simulink model "my_model"  (R2025b)
settings: Solver=FixedStepAuto  StartTime=0.0  StopTime=10.0  RelTol=1e-3
model workspace (MAT data in the model file):
  net = dlnetwork
  net.any.Version = 6
  net.any.LayerGraph = nnet.cnn.LayerGraph
  net.any.LayerGraph.any.Version = 1
  net.any.LayerGraph.any.Layers(1) = nnet.cnn.layer.FeatureInputLayer
  net.any.LayerGraph.any.Layers(1).any.Version = 2
  net.any.LayerGraph.any.Layers(1).any.Name = 'input_2'
  net.any.LayerGraph.any.Layers(1).any.InputSize = 5
  net.any.LayerGraph.any.Layers(1).any.Normalization = []
  net.any.LayerGraph.any.Layers(1).any.NormalizationDimension = 'auto'
  net.any.LayerGraph.any.Layers(1).any.SplitComplexInputs = 0
  net.any.LayerGraph.any.Layers(2) = nnet.cnn.layer.FullyConnectedLayer
  net.any.LayerGraph.any.Layers(2).any.Version = 3
  net.any.LayerGraph.any.Layers(2).any.Name = 'fc_'
  net.any.LayerGraph.any.Layers(2).any.InputSize = []
  net.any.LayerGraph.any.Layers(2).any.OutputSize = 128
  net.any.LayerGraph.any.Layers(2).any.Weights.Version = 2
  net.any.LayerGraph.any.Layers(2).any.Weights.Value = [0.145622700453 0.191488698125 1.34471386946e-25 0.192500352859 7.4865119314e-32 -1.01806771917e-35 0.0375644490123 0.00493536377326 0.148149654269 0.159106627107 3.70517046692e-39 0.172035083175 ... (640 elements, 128x5)]
  net.any.LayerGraph.any.Layers(2).any.Weights.LearnRateFactor = 1
  net.any.LayerGraph.any.Layers(2).any.Weights.L2Factor = 1
  net.any.LayerGraph.any.Layers(2).any.Weights.Initializer.Version = 1
  net.any.LayerGraph.any.Layers(2).any.Weights.Initializer.Class = 'nnet.internal.cnn.layer.learnable.initializer.Glorot'
  net.any.LayerGraph.any.Layers(2).any.Weights.Initializer.ConstructorArguments = {2, 1}
  net.any.LayerGraph.any.Layers(2).any.Bias.Version = 2
  net.any.LayerGraph.any.Layers(2).any.Bias.Value = [0.0191323123872 0.0192945022136 -0.0195418279618 0.0191192030907 -7.60889611815e-15 -9.2298071408e-09 0.223294004798 -0.0135857854038 -0.0391458682716 -0.0272029154003 -0.0109884552658 -0.0147490501404 ... (128 elements, 128x1)]
  net.any.LayerGraph.any.Layers(2).any.Bias.LearnRateFactor = 1
  net.any.LayerGraph.any.Layers(2).any.Bias.L2Factor = 0
  net.any.LayerGraph.any.Layers(2).any.Bias.Initializer.Version = 1
  net.any.LayerGraph.any.Layers(2).any.Bias.Initializer.Class = 'nnet.internal.cnn.layer.learnable.initializer.Zeros'
  net.any.LayerGraph.any.Layers(2).any.Bias.Initializer.ConstructorArguments = []
  net.any.LayerGraph.any.Layers(3) = nnet.cnn.layer.ReLULayer
  net.any.LayerGraph.any.Layers(3).any.Version = 1
  net.any.LayerGraph.any.Layers(3).any.Name = 're_lu_1'
  net.any.LayerGraph.any.Layers(4) = nnet.cnn.layer.FullyConnectedLayer
  net.any.LayerGraph.any.Layers(4).any.Version = 3
  net.any.LayerGraph.any.Layers(4).any.Name = 'fc_1_'
  net.any.LayerGraph.any.Layers(4).any.InputSize = []
  net.any.LayerGraph.any.Layers(4).any.OutputSize = 1
  net.any.LayerGraph.any.Layers(4).any.Weights.Version = 2
  net.any.LayerGraph.any.Layers(4).any.Weights.Value = [0.0540892928839 0.0813860446215 3.33540966394e-25 0.0615750215948 -1.09811353254e-30 -1.90163106556e-31 0.321531116962 -0.0607957392931 -0.1230366081 -0.0873386785388 4.04759007811e-38 -0.0916871502995 ... (128 elements, 1x128)]
  net.any.LayerGraph.any.Layers(4).any.Weights.LearnRateFactor = 1
  net.any.LayerGraph.any.Layers(4).any.Weights.L2Factor = 1
  net.any.LayerGraph.any.Layers(4).any.Weights.Initializer.Version = 1
  net.any.LayerGraph.any.Layers(4).any.Weights.Initializer.Class = 'nnet.internal.cnn.layer.learnable.initializer.Glorot'
  net.any.LayerGraph.any.Layers(4).any.Weights.Initializer.ConstructorArguments = {2, 1}
  net.any.LayerGraph.any.Layers(4).any.Bias.Version = 2
  net.any.LayerGraph.any.Layers(4).any.Bias.Value = 0.0196929574013
  net.any.LayerGraph.any.Layers(4).any.Bias.LearnRateFactor = 1
  net.any.LayerGraph.any.Layers(4).any.Bias.L2Factor = 0
  net.any.LayerGraph.any.Layers(4).any.Bias.Initializer.Version = 1
  net.any.LayerGraph.any.Layers(4).any.Bias.Initializer.Class = 'nnet.internal.cnn.layer.learnable.initializer.Zeros'
  net.any.LayerGraph.any.Layers(4).any.Bias.Initializer.ConstructorArguments = []
  net.any.LayerGraph.any.Connections = table
  net.any.LayerGraph.any.Connections.data = {{'input_2'; 'fc_'; 're_lu_1'}, {'fc_'; 're_lu_1'; 'fc_1_'}}
  net.any.LayerGraph.any.Connections.ndims = 2
  net.any.LayerGraph.any.Connections.nrows = 3
  net.any.LayerGraph.any.Connections.nvars = 2
  net.any.LayerGraph.any.Connections.varnames = {'Source', 'Destination'}
  net.any.LayerGraph.any.Connections.props.CustomProps = struct()
  net.any.LayerGraph.any.Connections.props.VariableCustomProps = struct()
  net.any.LayerGraph.any.Connections.props.versionSavedFrom = 5
  net.any.LayerGraph.any.Connections.props.minCompatibleVersion = 1
  net.any.LayerGraph.any.Connections.props.incompatibilityMsg = ''
  net.any.LayerGraph.any.Connections.props.VersionSavedFrom = 5
  net.any.LayerGraph.any.Connections.props.useVariableNamesOriginal = 0
  net.any.LayerGraph.any.Connections.props.useVariableNames2048 = 0
  net.any.LayerGraph.any.Connections.props.useDimensionNamesOriginal = 0
  net.any.LayerGraph.any.Connections.props.useDimensionNames2048 = 0
  net.any.LayerGraph.any.Connections.props.Description = ''
  net.any.LayerGraph.any.Connections.props.VariableNamesOriginal = {}
  net.any.LayerGraph.any.Connections.props.VariableNames2048 = {}
  net.any.LayerGraph.any.Connections.props.DimensionNames = {'Row', 'Variables'}
  net.any.LayerGraph.any.Connections.props.DimensionNamesOriginal = {}
  net.any.LayerGraph.any.Connections.props.DimensionNames2048 = {}
  net.any.LayerGraph.any.Connections.props.UserData = []
  net.any.LayerGraph.any.Connections.props.VariableDescriptions = {}
  net.any.LayerGraph.any.Connections.props.VariableUnits = {}
  net.any.LayerGraph.any.Connections.props.VariableContinuity = {}
  net.any.Initialized = 1
  net.any.SerializedQuantizationInfo.version = 1
  net.any.SerializedQuantizationInfo.data = containers.Map
  net.any.SerializedQuantizationInfo.data.serialization.keys = {}
  net.any.SerializedQuantizationInfo.data.serialization.values = {}
  net.any.SerializedQuantizationInfo.data.serialization.uniformity = 0
  net.any.SerializedQuantizationInfo.data.serialization.keyType = 'char'
  net.any.SerializedQuantizationInfo.data.serialization.valueType = 'any'
  net.any.ExampleInputs = {}
  net.any.OutputNames = {'fc_1_'}
  net.any.ExternalOutputNames = []
  net.any.ExternalInputNames = []
  net.any.RetainCustomInputNames = 1
  net.any.RetainCustomOutputNames = 1
libraries: dlconvfclib x2, dlactivationlib x1
settings Model: Creator=KantikaWongkasem  LastModifiedBy=KantikaWongkasem
settings OptimizationCC: DefaultParameterBehavior=Inlined  EnhancedBackFolding=on  PassReuseOutputArgsAs=Individual arguments  ZeroExternalMemoryAtStartup=off  ZeroInternalMemoryAtStartup=off  OptimizeBlockOrder=speed  DifferentSizesBufferReuse=on  OptimizationCustomize=off  EfficientTunableParamExpr=on
settings DebuggingCC: ParameterTunabilityLossMsg=error
settings SFSimCC: MATLABDynamicMemAlloc=off
settings RTWCC: SystemTargetFile=ert.tlc  TemplateMakefile=ert_default_tmf  Description=Embedded Coder
settings CodeAppCC: ForceParamTrailComments=on  IgnoreCustomStorageClasses=off  OperatorAnnotations=on  SimulinkDataObjDesc=on  SFDataObjDesc=on  InsertBlockDesc=on
settings ERTTargetCC: ERTCustomFileTemplate=example_file_process.tlc  TargetLangStandard=C99 (ISO)  GenerateSampleERTMain=on

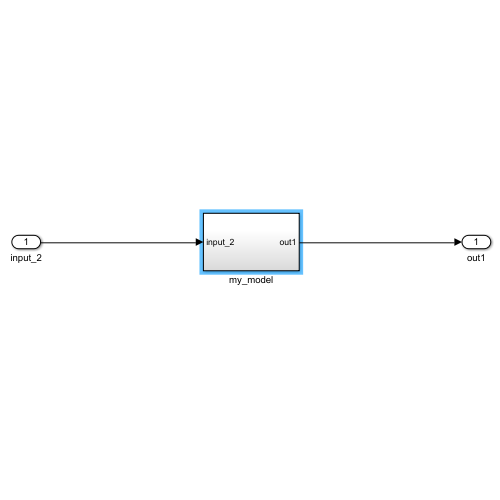
[thumbnail: Simulink's stored preview of the top-level diagram]
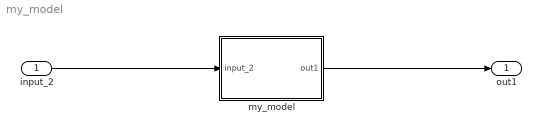
== system my_model ==
  input_2 : Inport  PortDimensions=[5]
  my_model : Subsystem
  out1 : Outport
  wires:
  input_2/1 -> my_model/1(input_2)
  my_model/1(out1) -> out1/1

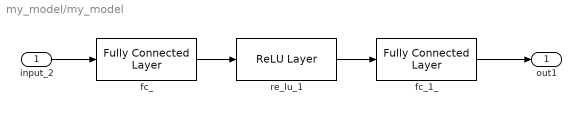
== system my_model/my_model ==
  input_2 : Inport  PortDimensions=[5]
  fc_ : dlconvfclib/Fully Connected Layer  Layer=net.Layers(2)  OutMin=[]  OutMax=[]  WeightsDataTypeStr=Inherit: Inherit via back propagation  WeightsMin=[]  WeightsMax=[]  BiasDataTypeStr=Inherit: Inherit via back propagation  BiasMin=[]  BiasMax=[]  AccumMin=[]  AccumMax=[]  InternalRndMeth=Floor  InternalSaturateOnIntegerOverflow=off  SampleTime=-1
      settings: DataFormat=C
  fc_1_ : dlconvfclib/Fully Connected Layer  Layer=net.Layers(4)  OutMin=[]  OutMax=[]  WeightsDataTypeStr=Inherit: Inherit via back propagation  WeightsMin=[]  WeightsMax=[]  BiasDataTypeStr=Inherit: Inherit via back propagation  BiasMin=[]  BiasMax=[]  AccumMin=[]  AccumMax=[]  InternalRndMeth=Floor  InternalSaturateOnIntegerOverflow=off  SampleTime=-1
      settings: DataFormat=C
  re_lu_1 : dlactivationlib/ReLU Layer  OutMin=[]  OutMax=[]  SampleTime=-1
  out1 : Outport
  wires:
  fc_/1 -> re_lu_1/1
  re_lu_1/1 -> fc_1_/1
  fc_1_/1 -> out1/1
  input_2/1 -> fc_/1
